simulink model "uwm_client"  (R2022b)
settings: Solver=VariableStepAuto  StartTime=0.0  StopTime=10.0  RelTol=1e-3
undefined symbols (not defined in the file): f
libraries: instrumentlib x2
settings Model: Creator=saigon  LastModifiedBy=saigon

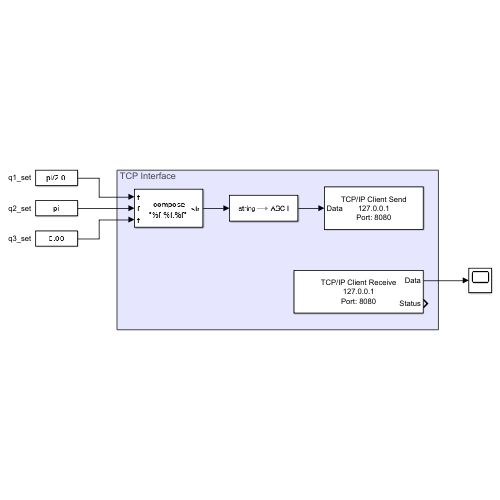
[thumbnail: Simulink's stored preview of the top-level diagram]
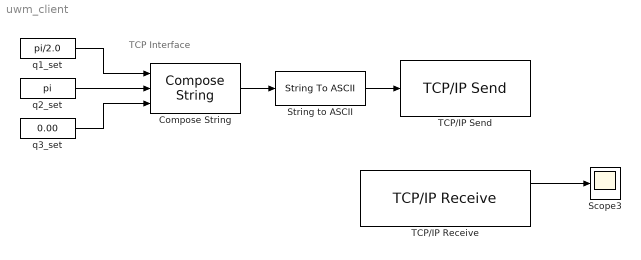
== system uwm_client ==
  note: TCP Interface
  Compose String : ComposeString  Format="\"%f,%f,%f\""
  Scope3 : Scope
  String to ASCII : StringToASCII
  TCP/IP Receive : instrumentlib/TCP//IP Receive  Host=127.0.0.1  Port=8080  DataSize=[ 3,1 ]  DataType=ASCII  ASCIIFormatting=%f,%f,%f  Terminator=LF  CustomTerminator=10  ByteOrder=big-endian  EnableBlockingMode=off  Timeout=10  SampleTime=0.01  SimulateUsing=Interpreted execution
  TCP/IP Send : instrumentlib/TCP//IP Send  Host=127.0.0.1  Port=8080  ByteOrder=big-endian  EnableBlockingMode=off  Timeout=10  TransferDelay=on  SimulateUsing=Interpreted execution
  q1_set : Constant  Value=pi/2.0
  q2_set : Constant  Value=pi
  q3_set : Constant  Value=0.00
  wires:
  String to ASCII/1 -> TCP/IP Send/1
  Compose String/1 -> String to ASCII/1
  q1_set/1 -> Compose String/1
  q2_set/1 -> Compose String/2
  q3_set/1 -> Compose String/3
  TCP/IP Receive/1 -> Scope3/1
